simulink model "Control_SwitchCase"  (R2015b)
settings: Solver=VariableStepAuto  StartTime=0.0  StopTime=10.0  RelTol=1e-3
StartFcn:
  | open_scope
libraries: simulink x1
settings Model: Creator=LUBO  LastModifiedBy=LUBO

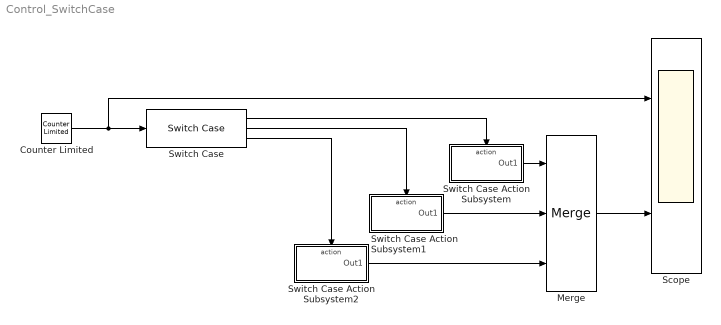
== system Control_SwitchCase ==
  Counter Limited : simulink/Sources/Counter Limited  uplimit=8  tsamp=0.2
  Merge : Merge  Inputs=3
  Scope : Scope  NumInputPorts=2
  Switch Case : SwitchCase  CaseConditions={[1 2 3],[5 6 7 8]}
  Switch Case Action Subsystem : Subsystem  TreatAsAtomicUnit=on
  Switch Case Action Subsystem1 : Subsystem  TreatAsAtomicUnit=on
  Switch Case Action Subsystem2 : Subsystem  TreatAsAtomicUnit=on
  wires:
  Switch Case/1 -> Switch Case Action Subsystem/Action
  Switch Case/2 -> Switch Case Action Subsystem1/Action
  Switch Case/3 -> Switch Case Action Subsystem2/Action
  Switch Case Action Subsystem/1(Out1) -> Merge/1
  Switch Case Action Subsystem1/1(Out1) -> Merge/2
  Switch Case Action Subsystem2/1(Out1) -> Merge/3
  Counter Limited/1 -> Switch Case/1, Scope/1
  Merge/1 -> Scope/2

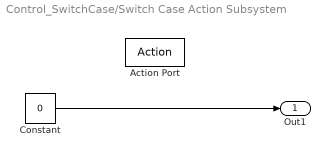
== system Control_SwitchCase/Switch Case Action Subsystem ==
  Action Port : ActionPort  ActionType=case
  Constant : Constant  Value=0
  Out1 : Outport
  wires:
  Constant/1 -> Out1/1

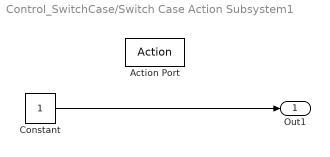
== system Control_SwitchCase/Switch Case Action Subsystem1 ==
  Action Port : ActionPort  ActionType=case
  Constant : Constant
  Out1 : Outport
  wires:
  Constant/1 -> Out1/1

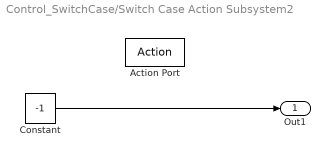
== system Control_SwitchCase/Switch Case Action Subsystem2 ==
  Action Port : ActionPort  ActionType=default
  Constant : Constant  Value=-1
  Out1 : Outport
  wires:
  Constant/1 -> Out1/1
